simulink model "Lab4_MSK"  (Simulink 10.2)
settings: Solver=VariableStepAuto  StartTime=0.0  StopTime=10  RelTol=1e-3
libraries: commsequence2 x1, commseqgen3 x1, dspspect3 x1, simulink x1, commutil2 x1
settings Model: Creator=Newtr  LastModifiedBy=Newtr
settings DataIOCC: SaveFormat=Dataset  SignalLoggingSaveFormat=Dataset  ReturnWorkspaceOutputs=on
settings OptimizationCC: LifeSpan=auto
settings DebuggingCC: UnderspecifiedInitializationDetection=Simplified  MergeDetectMultiDrivingBlocksExec=error  FcnCallInpInsideContextMsg=error  SFUnexpectedBacktrackingDiag=error  SFNoUnconditionalDefaultTransitionDiag=error  SFExecutionAtInitializationDiag=warning  ArithmeticOperatorsInVariantConditions=error
settings HardwareCC: ProdBitPerPointer=64  ProdBitPerSizeT=64  ProdBitPerPtrDiffT=64  ProdLargestAtomicFloat=Float  ProdIntDivRoundTo=Zero  ProdEndianess=LittleEndian  ProdWordSize=64  ProdHWDeviceType=Intel->x86-64 (Windows64)
settings ModelReferenceCC: PropagateSignalLabelsOutOfModel=on
settings SFSimCC: SimUseLocalCustomCode=on  CustomCodeUndefinedFunction=FilterOut
settings RTWCC: RTWUseLocalCustomCode=on
settings CodeAppCC: StateflowObjectComments=off
settings GRTTargetCC: TargetLangStandard=C99 (ISO)  CombineOutputUpdateFcns=on  GRTInterface=off
settings ConfigComp: CovMetricSettings=dwe  CovSaveCumulativeToWorkspaceVar=off  CovSaveSingleToWorkspaceVar=off  CovExternalEMLEnable=on

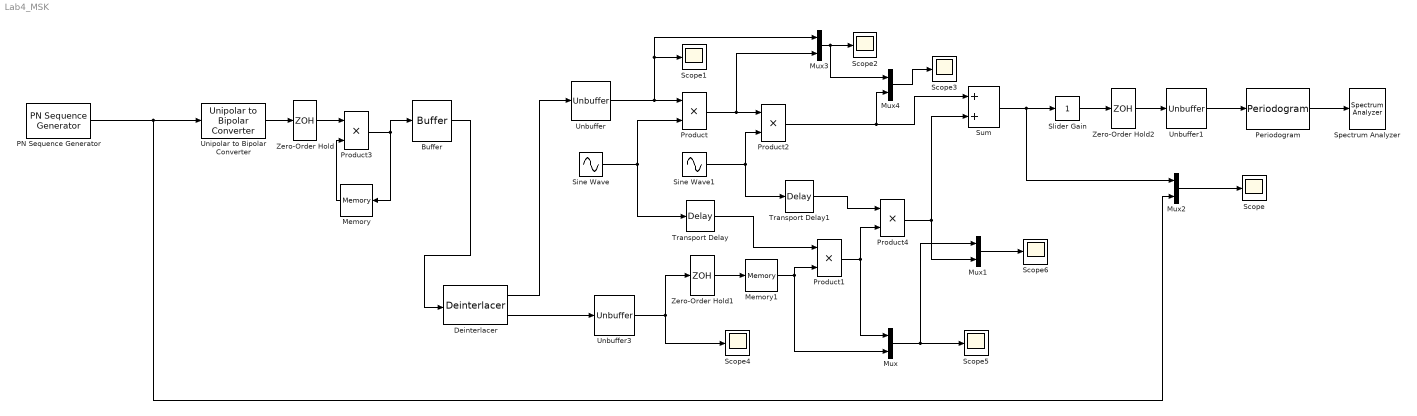
== system Lab4_MSK ==
  Buffer : Buffer  N=2  OutputFrames=off
  Deinterlacer : commsequence2/Deinterlacer
      settings: SourceProductBaseCode=CM
  Memory : Memory  InitialCondition=1  InheritSampleTime=on
  Memory1 : Memory  InheritSampleTime=on
  Mux{,1..4} (5 alike) : Mux  Inputs=2
  PN Sequence Generator : commseqgen3/PN Sequence Generator  poly='z^6 + z + 1'  ini_sta=[0 0 0 0 0 1]  outBitMaskSource=Dialog parameter  shift=0  outVarSiz=off  maxOutSizeMode=Dialog parameter  maxOutSize=[10 1]  Ts=1/1200  sampPerFrame=1  reset=off  bitPackedOutputs=off  outDataType=double  numPackedBits=8  bitPackDataSigned=off  bitPackedOutDType=double
  Periodogram : dspspect3/Periodogram  measurement=Power spectral density  wintype=Hamming  Rs=50  beta=5  winsamp=Symmetric  FFTImplementation=Auto  inheritFFT=off  fftsize=256  navg=4  inheritTs=on  Ts=1
      settings: SourceProductBaseCode=DS
  Product{,1..4} (5 alike) : Product
  Scope{,1..6} (7 alike) : Scope
  Sine Wave : Sin  Frequency=600*pi  Phase=-pi  SampleTime=0
  Sine Wave1 : Sin  Frequency=76000*pi  SampleTime=0
  Slider Gain : simulink/Math Operations/Slider Gain  gain=1  low=0  high=2
  Spectrum Analyzer : SpectrumAnalyzer
  Sum : Sum
  Transport Delay : TransportDelay  DelayTime=1/1200
  Transport Delay1 : TransportDelay  DelayTime=3/38000/4
  Unbuffer : Unbuffer
  Unbuffer1 : Unbuffer
  Unbuffer3 : Unbuffer
  Unipolar to Bipolar Converter : commutil2/Unipolar to Bipolar Converter  M=2  polarity=Positive  dataType=Inherit via internal rule
  Zero-Order Hold : ZeroOrderHold  SampleTime=1/1200
  Zero-Order Hold1 : ZeroOrderHold  SampleTime=1/1200
  Zero-Order Hold2 : ZeroOrderHold  SampleTime=1/14000/3
  wires:
  PN Sequence Generator/1 -> Unipolar to Bipolar Converter/1, Mux2/2
  Unipolar to Bipolar Converter/1 -> Zero-Order Hold/1
  Zero-Order Hold/1 -> Product3/1
  Product3/1 -> Memory/1, Buffer/1
  Buffer/1 -> Deinterlacer/1
  Memory/1 -> Product3/2
  Deinterlacer/2 -> Unbuffer3/1
  Deinterlacer/1 -> Unbuffer/1
  Product/1 -> Mux3/2, Product2/1
  Unbuffer3/1 -> Zero-Order Hold1/1, Scope4/1
  Zero-Order Hold1/1 -> Memory1/1
  Memory1/1 -> Product1/2, Mux/2
  Product1/1 -> Product4/2, Mux/1
  Mux/1 -> Mux1/1, Scope5/1
  Mux1/1 -> Scope6/1
  Mux2/1 -> Scope/1
  Transport Delay/1 -> Product1/1
  Sine Wave/1 -> Product/2, Transport Delay/1
  Sine Wave1/1 -> Product2/2, Transport Delay1/1
  Transport Delay1/1 -> Product4/1
  Unbuffer/1 -> Mux3/1, Scope1/1, Product/1
  Mux3/1 -> Mux4/1, Scope2/1
  Product4/1 -> Mux1/2, Sum/2
  Product2/1 -> Mux4/2, Sum/1
  Mux4/1 -> Scope3/1
  Sum/1 -> Mux2/1, Slider Gain/1
  Slider Gain/1 -> Zero-Order Hold2/1
  Zero-Order Hold2/1 -> Unbuffer1/1
  Unbuffer1/1 -> Periodogram/1
  Periodogram/1 -> Spectrum Analyzer/1
